simulink model "baby_model"  (R2024b)
settings: Solver=ode5  StartTime=0.0  StopTime=3  FixedStep=1/1000  RelTol=1e-3
values from neighbouring files (symbols this model uses):
  N = 50    [save_hankel_data_gemini.m]
  T_ini = 20    [save_hankel_data_gemini.m]
  Uf = U_hankel(T_ini+1:end, :)    [save_hankel_data_gemini.m]
  Up = U_hankel(1:T_ini, :)    [save_hankel_data_gemini.m]
  Yf = Y_hankel(T_ini+1:end, :)    [save_hankel_data_gemini.m]
  Yp = Y_hankel(1:T_ini, :)    [save_hankel_data_gemini.m]
libraries: simulink x3, slpidlib x1
settings Model: Creator=scherg  LastModifiedBy=scherg

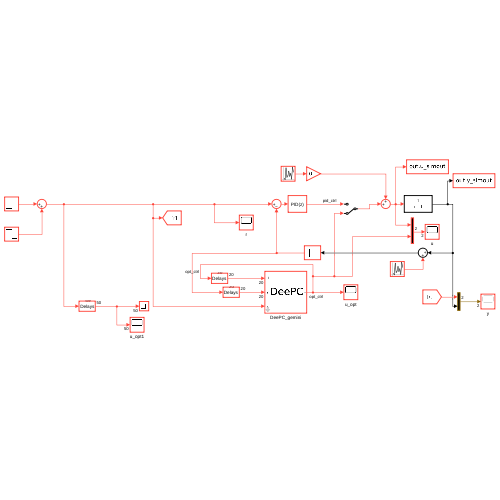
[thumbnail: Simulink's stored preview of the top-level diagram]
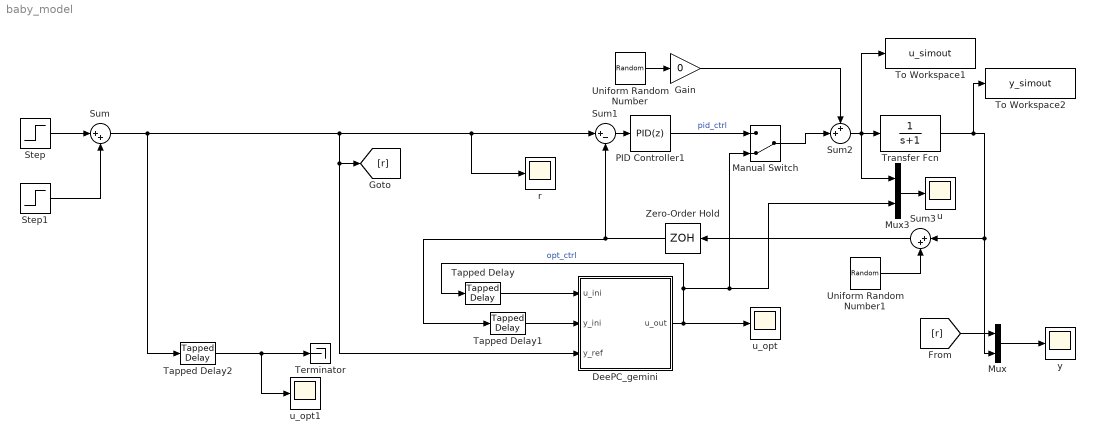
== system baby_model ==
  DeePC_gemini : MATLAB Function  TreatAsAtomicUnit=on  mask{Up=Up, Yp=Yp, Uf=Uf, Yf=Yf, q=400, r=1, lambda=1e-4, u_limit=4.0}
      mask prompts: q "Higher Bandwidth Increase Q"; r "Better Smoothness Increase R"; lambda "larger lambda makes the controller more robust to disturbances and noise"; u_limit "Control signal limit (+-)"
  Gain : Gain  Gain=0
  Manual Switch : ManualSwitch  CurrentSetting=0
  Mux : Mux  Inputs=2
  Mux3 : Mux  Inputs=2
  PID Controller1 : slpidlib/PID Controller  Controller=PID  Form=Parallel  TimeDomain=Discrete-time  UseExternalTs=off  SampleTime=1/1000  IntegratorMethod=Forward Euler  FilterMethod=Forward Euler  ControllerParametersSource=internal  P=1  I=0  UseKiTs=off  D=0  UseExternalDerivativeSource=off  N=100  UseFilter=on  TunerSelectOption=Transfer Function Based (PID Tuner App)  InitialConditionSource=internal  InitialConditionForIntegrator=0  InitialConditionForFilter=0  DifferentiatorICPrevScaledInput=0  ExternalReset=none  TrackingMode=off  Kt=1  LimitOutput=off  SatLimitsSource=internal  UpperSaturationLimit=inf  LowerSaturationLimit=-inf  LinearizeAsGain=on  AntiWindupMode=none  Kb=1  LimitIntegrator=off  UpperIntegratorSaturationLimit=inf  LowerIntegratorSaturationLimit=-inf  POutMin=[]  POutMax=[]  IOutMin=[]  IOutMax=[]  DOutMin=[]  DOutMax=[]  NOutMin=[]  NOutMax=[]  SumOutMin=[]  SumOutMax=[]  SaturationOutMin=[]  SaturationOutMax=[]  PParamMin=[]  PParamMax=[]  IParamMin=[]  IParamMax=[]  DParamMin=[]  DParamMax=[]  NParamMin=[]  NParamMax=[]  KbParamMin=[]  KbParamMax=[]  KtParamMin=[]  KtParamMax=[]  KbOutMin=[]  KbOutMax=[]  KtOutMin=[]  KtOutMax=[]  IntegratorOutMin=[]  IntegratorOutMax=[]  FilterOutMin=[]  FilterOutMax=[]  SumI1OutMin=[]  SumI1OutMax=[]  SumI2OutMin=[]  SumI2OutMax=[]  SumI3OutMin=[]  SumI3OutMax=[]  SumI4OutMin=[]  SumI4OutMax=[]  SumDOutMin=[]  SumDOutMax=[]  DifferentiatorOutMin=[]  DifferentiatorOutMax=[]  FilterDiffOutCoefMin=[]  FilterDiffOutCoefMax=[]  ReciprocalOutMin=[]  ReciprocalOutMax=[]  SumDenOutMin=[]  SumDenOutMax=[]  SumNumOutMin=[]  SumNumOutMax=[]  DivideOutMin=[]  DivideOutMax=[]  UdiffTsProdOutMin=[]  UdiffTsProdOutMax=[]  NTsProdOutMin=[]  NTsProdOutMax=[]  UintegralTsProdOutMin=[]  UintegralTsProdOutMax=[]  UngainTsProdOutMin=[]  UngainTsProdOutMax=[]  ClampingZeroOutDataTypeStr=Inherit: Inherit via back propagation  ClampingZeroOutMin=[]  ClampingZeroOutMax=[]  FilterDenConstantOutDataTypeStr=Inherit: Inherit via back propagation  FilterDenConstantOutMin=[]  FilterDenConstantOutMax=[]  PCopyOutDataTypeStr=Inherit: Inherit via back propagation  PCopyOutMin=[]  PCopyOutMax=[]  NCopyOutDataTypeStr=Inherit: Inherit via back propagation  NCopyOutMin=[]  NCopyOutMax=[]  IntegratorContinuousStateAttributes=''  IntegratorStateMustResolveToSignalObject=off  IntegratorRTWStateStorageClass=Auto  FilterContinuousStateAttributes=''  FilterStateMustResolveToSignalObject=off  FilterRTWStateStorageClass=Auto  ParallelPVariant=InternalParameters  IdealPVariant=Disabled  IVariant=InternalParameters  DVariant=InternalParameters  IntegratorVariant=Discrete  SatVariant=Disabled  AWVariant=Passthrough  PCopyVariant=Disabled  TRVariant=Disabled  FdbkBlocksVariant=Forward  IdealPFdbkVariant=Disabled  SatFdbkVariant=Disabled  DerivativeFilterVariant=ForwardEulerFilter  NVariant=InternalParameters  NCopyVariant=Disabled  FilterICVariant=InternalICsFilter  IntegratorICVariant=InternalICs  ExternalResetVariant=Disabled  TRSumVariant=Passthrough  SumFdbkVariant=Disabled  SumVariant=Sum_PID  TsampFilterVariant=InternalTs  TsampNgainVariant=Passthrough  TsampIntegralVariant=Disabled_SignalSpec  ExternalSaturationOutDataTypeStr=Inherit: Same as second input  DerivativeSourceVariant=ErrorSignal  PreIntVariant=InternalPreInt
  Step : Step  SampleTime=1/1000
  Step1 : Step  Time=2  After=-2  SampleTime=1/1000
  Sum : Sum  Inputs=|++
  Sum1 : Sum  Inputs=|+-
  Sum2 : Sum  Inputs=++|
  Sum3 : Sum  Inputs=|++
  Tapped Delay : simulink/Discrete/Tapped Delay  vinit=0.0  samptime=1/1000  NumDelays=T_ini  DelayOrder=Oldest  includeCurrent=off
  Tapped Delay1 : simulink/Discrete/Tapped Delay  vinit=0.0  samptime=1/1000  NumDelays=T_ini  DelayOrder=Oldest  includeCurrent=off
  Tapped Delay2 : simulink/Discrete/Tapped Delay  vinit=0.0  samptime=1/1000  NumDelays=N-1  DelayOrder=Oldest  includeCurrent=on
  Terminator : Terminator
  To Workspace1 : ToWorkspace  VariableName=u_simout  SaveFormat=Structure With Time  SampleTime=-1
  To Workspace2 : ToWorkspace  VariableName=y_simout  SaveFormat=Structure With Time  SampleTime=-1
  Transfer Fcn : TransferFcn  Denominator=[1 1]
  Uniform Random Number : UniformRandomNumber  Minimum=-0.1  Maximum=0.1  SampleTime=1/1000
  Uniform Random Number1 : UniformRandomNumber  Minimum=-0.1  Maximum=0.1  SampleTime=1/1000
  Zero-Order Hold : ZeroOrderHold  SampleTime=1/1000
  r : Scope
  u : Scope
  u_opt : Scope
  u_opt1 : Scope
  y : Scope
  wires:
  Sum1/1 -> PID Controller1/1
  PID Controller1/1 -> Manual Switch/1  "pid_ctrl"
  Transfer Fcn/1 -> To Workspace2/1, Mux/2, Sum3/1
  DeePC_gemini/1(u_out) -> Manual Switch/2, Mux3/2, Tapped Delay/1, u_opt/1  "opt_ctrl"
  Mux3/1 -> u/1
  Zero-Order Hold/1 -> Tapped Delay1/1, Sum1/2
  Sum2/1 -> To Workspace1/1, Mux3/1, Transfer Fcn/1
  Uniform Random Number/1 -> Gain/1
  Step/1 -> Sum/1
  Gain/1 -> Sum2/1
  Tapped Delay/1 -> DeePC_gemini/1(u_ini)
  Tapped Delay1/1 -> DeePC_gemini/2(y_ini)
  Step1/1 -> Sum/2
  Tapped Delay2/1 -> Terminator/1, u_opt1/1
  Sum/1 -> DeePC_gemini/3(y_ref), [r], Sum1/1, r/1, Tapped Delay2/1
  Manual Switch/1 -> Sum2/2
  [r] -> Mux/1
  Mux/1 -> y/1
  Uniform Random Number1/1 -> Sum3/2
  Sum3/1 -> Zero-Order Hold/1

== matlab function baby_model/DeePC_gemini ==
  data: u_ini input size=[T_ini 1]; u_out output size=[1 1]; y_ini input size=[T_ini 1]; y_ref input size=[1 1]; Up parameter; Yp parameter; Uf parameter; Yf parameter; q parameter; r parameter; lambda parameter; u_limit parameter
function u_out = deepc_controller(u_ini, y_ini, y_ref, Up, Yp, Uf, Yf, q, r, lambda, u_limit)

    % u_ini: [Tini*m x 1] 
    % y_ini: [Tini*p x 1]
    % y_ref: [N*p x 1]
    % Up, Uf, Yp, Yf: Pre-partitioned Hankel matrices from offline data

    % --- Persistent Variables for Speed ---
    persistent G_mat x0_warm first_run m p N Tini u_prev u_f_sol Q R du_max du_min A_cons I_vec S
    
    % --- Initialization (t = 0) ---
    if isempty(first_run)
        [row_Up, ~] = size(Up);
        [row_Uf, ~] = size(Uf);
        [row_Yp, ~] = size(Yp);
        [row_Yf, ~] = size(Yf);
        
        m = 1; % Adjust to your number of inputs
        p = 1; % Adjust to your number of outputs
        Tini = row_Up / m;
        N = row_Uf / m;

        % Compute the "Image" of the data (the G matrix)
        % This projects the relationship into the input/output space
        % g_fixed = [Up; Yp; Uf] pinv * [u_ini; y_ini; u_f]
        % We pre-calculate the fundamental mapping:
        % --- 1. Disturbance Rejection Knob (Lambda) ---
        % lambda = 1e-4; % Increase this to 1e-2 if system is too "twitchy"
        H_offline = [Up; Yp; Uf];
        % Regularized pseudo-inverse
        H_pseudo = (H_offline' * H_offline + lambda * eye(size(H_offline,2))) \ H_offline';
        % H_pseudo = pinv([Up; Yp; Uf]); 
        G_mat = Yf * H_pseudo; 

        u_f_sol = zeros(N*m+1, 1); % plus slack

        % --- The Incremental Logic ---
        % u_f(k) = u(t-1) + sum_{i=1}^{k} delta_u(i)
        % We create a Summation Matrix 'S' to relate delta_u to absolute u_f
        % u_f = S * delta_u + I_vec * u_prev
        S = tril(ones(N*m)); 
        I_vec = ones(N*m, 1);
        A_cons = [S, -ones(N*m, 1); -S, -ones(N*m, 1)]; % Inequality matrix for absolute saturation with Slack Buffer

        % --- Weights (Tune these!) ---
        Q = eye(size(Yf, 1)) * q;  % Output tracking weight
        R = eye(size(Uf, 1)) * r;    % Control effort weight

        % --- Constraints ---
        % Example: du_min <= u_f <= du_max % Lower bound for slack: must be >= 0
        du_max = [3 * ones(N*m, 1); inf]; 
        du_min = [-3 * ones(N*m, 1); 0];
        
        % Initialize warm start vector for u_f (size N*m)
        x0_warm = zeros(N*m+1, 1);
        u_prev = 0;              % To track the absolute u applied
        first_run = 1;
        u_out = 0;
        return;
    end

    % Slack Weight (S_w): Must be MUCH larger than Q to keep constraints "hard"
    % until they absolutely must be broken.
    S_w = 1e6;

    % --- Construct Reduced QP ---
    % Standard DeePC: min ||Yf*g - y_ref||^2_Q + ||Uf*g||^2_R
    % Reduced: We express Yf*g as a function of u_f and initial conditions
    
    % Split the pre-calculated projection for the current [u_ini; y_ini]
    % Yf*g = G1*u_ini + G2*y_ini + G3*u_f
    G_const = G_mat(:, 1:size(Up,1)+size(Yp,1));
    G_v = G_mat(:, size(Up,1)+size(Yp,1)+1:end);
    % Fixed part of the prediction based on past data
    % y_fixed = G_const * [u_ini; y_ini];
    y_fixed = G_const * [u_ini; y_ini] + G_v * I_vec * u_prev;

    y_ref_vec = y_ref*ones(N,1);

    % Quadratic Programming form: 0.5*u_f'*H_qp*u_f + f_qp'*u_f
    M = G_v * S;
    % Augmented Hessian: H_total = [H_qp, 0; 0, S_w]
    H_qp_core = 2 * (M' * Q * M + R);
    H_qp = blkdiag(H_qp_core, S_w);
    % Augmented f: f_total = [f_qp; 0]
    f_qp_core = 2 * M' * Q * (y_fixed - y_ref_vec);
    f_qp = [f_qp_core; 0];
    
    % Force symmetry to satisfy quadprog
    H_qp = (H_qp + H_qp') / 2;

    % --- 2. Absolute Saturation Limits ---
    % u_limit = 4.0; % Example: throttle/steering limit
    % b_cons changes every step because it depends on u_prev
    b_cons = [u_limit * I_vec - I_vec * u_prev; 
              u_limit * I_vec + I_vec * u_prev];
    
    
    % --- Solver Options ---
    % 'active-set' is required for Simulink Code Generation
    opts = optimoptions('quadprog', 'Display', 'off', 'Algorithm', 'active-set');
    
    % Call Solver with Warm Start (x0_warm)
    coder.extrinsic('quadprog');
    
    exitflag = 0;
    
    [u_f_sol, ~, exitflag] = quadprog(H_qp, f_qp, A_cons, b_cons, [], [], du_min, du_max, x0_warm, opts);

    % --- Output and Warm Start Update ---
    if exitflag > 0
        % Apply the first control action
        delta_u_now = u_f_sol(1); %:m);
        u_out = u_prev + delta_u_now;
        
        % Update for next step
        u_prev = u_out;
        % Update Warm Start for next iteration (Shift-and-append)
        % We shift the solution one step and pad with the last value
        x0_warm = [u_f_sol(m+1:end-1); 0; u_f_sol(end)]; % Shift delta_u, keep slack %(m+1:end); u_f_sol(end-m+1:end)];
    else
        % If optimization fails, fallback to previous or zero
        u_out = u_prev;
    end
end

%     % u_ini: [T_ini x 1] vector of recent inputs
%     % y_ini: [T_ini x 1] vector of recent outputs
%     % y_ref: [N x 1] vector of desired future outputs
%     u_out = 0; % Pre-allocate so Simulink knows the type
%     persistent last_u H_mat f_vec Aeq n_vars x0
%     if isempty(last_u)
%         last_u = 0; 
%     end
% 
%     % Decision variable for quadprog: [g; sigma]
%     % We use the g-vector to span the signal space and sigma to handle noise
%     num_columns = size(Up, 2);
%     num_sigma = size(Yp, 1);
% 
%     % --- Cost Function Formulation ---
%     % We want to minimize: ||Yf*g - y_ref||^2_Q + ||Uf*g||^2_R + L_g*||g||^2 + L_s*||sigma||^2
%     % 0.5 * z' * H_mat * z + f_vec' * z
% 
%     if isempty(H_mat)
%         H_mat = blkdiag(2*(Yf'*Q*Yf + Uf'*R*Uf + lambda_g*eye(num_columns)), 2*lambda_sigma*eye(num_sigma));
%         H_mat = (H_mat + H_mat') / 2; % Ensure perfect symmetry for the solver
%         f_vec = [(-2*y_ref'*Q*Yf)'; zeros(num_sigma, 1)];
% 
%         % --- Equality Constraints ---
%         % [Up; Yp]*g + [0; sigma] = [u_ini; y_ini]
%         Aeq = [Up, zeros(size(Up, 1), num_sigma); 
%                Yp, eye(num_sigma)];
% 
%         n_vars = size(H_mat, 1);
%         x0 = zeros(n_vars, 1);
%     end
%     beq = [u_ini; y_ini];
% 
%     % --- Solving (Using interior-point for speed) ---
%     opts = optimoptions('quadprog', 'Display', 'off', 'Algorithm', 'active-set');
%     % Define the number of decision variables (usually g = size(U_p, 2))
% 
%     z_opt = quadprog(H_mat, f_vec, [], [], Aeq, beq, [], [], x0, opts);
% 
%     if isempty(z_opt)
%         u_out = last_u; % Fallback if optimization fails
%     else
%         g_opt = z_opt(1:num_columns);
%         u_future = Uf * g_opt;
%         u_out = u_future(1); % Apply first step (Receding Horizon)
%         last_u = u_out;
%     end
% end
